simulink model "model"  (R2023b)
settings: Solver=VariableStepAuto  StartTime=0.0  StopTime=10.0  RelTol=1e-3
values from neighbouring files (symbols this model uses):
  A = sqrt(2)*wc    [main.m]
  B = wc^2    (= 157.913670417)    [main.m]
  LPF1 = tf(LPF1_num,LPF1_den)    [main.m]
  LPF2 = tf(LPF2_num,LPF2_den)    [main.m]
  LPF3 = tf(LPF3_num,LPF3_den)    [main.m]
  sysc = tf([K*wn^2],[1,2*zeta*wn,wn^2])*tf([1],[0.3,1])    [main.m]
  sysc2 = tf([-K*wn^2],[1,2*zeta*wn,wn^2])*tf([1],[0.1,1])    [main.m]
  Ts = 0.01    [main.m]
libraries: SignalEditorBlockLib x1
settings Model: Creator=block  LastModifiedBy=block
settings DataIOCC: ReturnWorkspaceOutputs=off

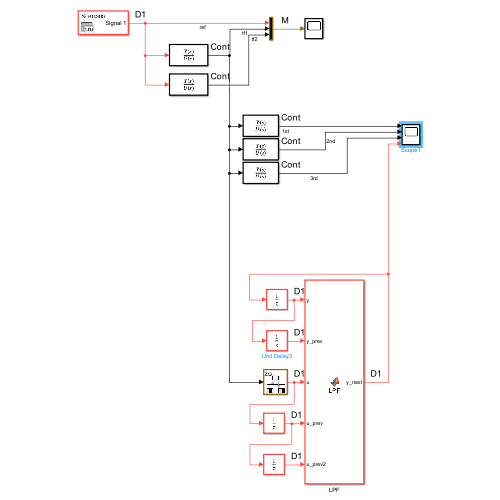
[thumbnail: Simulink's stored preview of the top-level diagram]
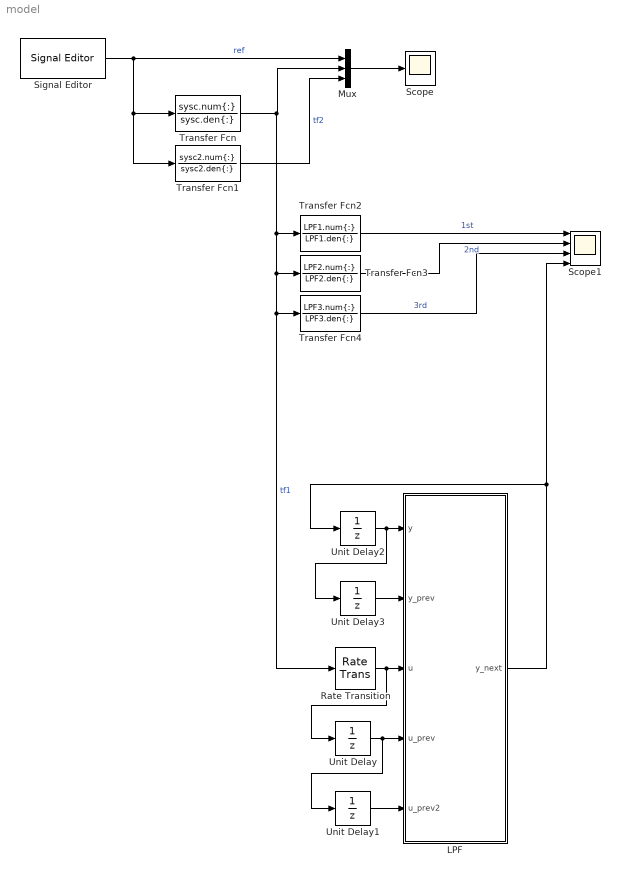
== system model ==
  LPF : MATLAB Function  TreatAsAtomicUnit=on
  Mux : Mux  Inputs=3
  Rate Transition : RateTransition  OutPortSampleTime=Ts
  Scope : Scope
  Scope1 : Scope  NumInputPorts=4
  Signal Editor : SignalEditorBlockLib/Signal Editor  FileName=input.mat  ActiveScenario=Scenario  ActiveSignal=Signal 1  IsBus=off  OutputBusObjectStr=Bus: BusObject  SampleTime=0.01  ZeroCross=off  OutputAfterFinalValue=Setting to zero  Unit=inherit  PreserveSignalName=on  ApplySigPropsToAllScenarios=on  ApplySigPropsToAllSignals=off
  Transfer Fcn : TransferFcn  Numerator=sysc.num{:}  Denominator=sysc.den{:}
  Transfer Fcn1 : TransferFcn  Numerator=sysc2.num{:}  Denominator=sysc2.den{:}
  Transfer Fcn2 : TransferFcn  Numerator=LPF1.num{:}  Denominator=LPF1.den{:}
  Transfer Fcn3 : TransferFcn  Numerator=LPF2.num{:}  Denominator=LPF2.den{:}
  Transfer Fcn4 : TransferFcn  Numerator=LPF3.num{:}  Denominator=LPF3.den{:}
  Unit Delay{,1..3} (4 alike) : UnitDelay  SampleTime=-1  HasFrameUpgradeWarning=on
  wires:
  Signal Editor/1 -> Mux/1, Transfer Fcn1/1, Transfer Fcn/1  "ref"
  Transfer Fcn/1 -> Transfer Fcn2/1, Rate Transition/1, Transfer Fcn4/1, Transfer Fcn3/1, Mux/2  "tf1"
  Transfer Fcn1/1 -> Mux/3  "tf2"
  Mux/1 -> Scope/1
  Transfer Fcn3/1 -> Scope1/2  "2nd"
  Transfer Fcn4/1 -> Scope1/3  "3rd"
  Transfer Fcn2/1 -> Scope1/1  "1st"
  Rate Transition/1 -> Unit Delay/1, LPF/3(u)
  LPF/1(y_next) -> Scope1/4, Unit Delay2/1
  Unit Delay2/1 -> Unit Delay3/1, LPF/1(y)
  Unit Delay3/1 -> LPF/2(y_prev)
  Unit Delay/1 -> Unit Delay1/1, LPF/4(u_prev)
  Unit Delay1/1 -> LPF/5(u_prev2)

== matlab function model/LPF ==
  data: y input; y_prev input; u input; u_prev input; u_prev2 input; y_next output; A parameter; B parameter; Ts parameter
function y_next = LPF(y,y_prev,u,u_prev,u_prev2,A,B, Ts)
    y_next = (2-A*Ts)*y-(1-A*Ts+B*Ts*Ts)*y_prev+u-2*u_prev+u_prev2;
end
